simulink model "task1-1"  (R2016a)
settings: Solver=VariableStepAuto  StartTime=0.0  StopTime=10.0  RelTol=1e-3
libraries: simulink x1
settings Model: Creator=Misachu  LastModifiedBy=Misachu

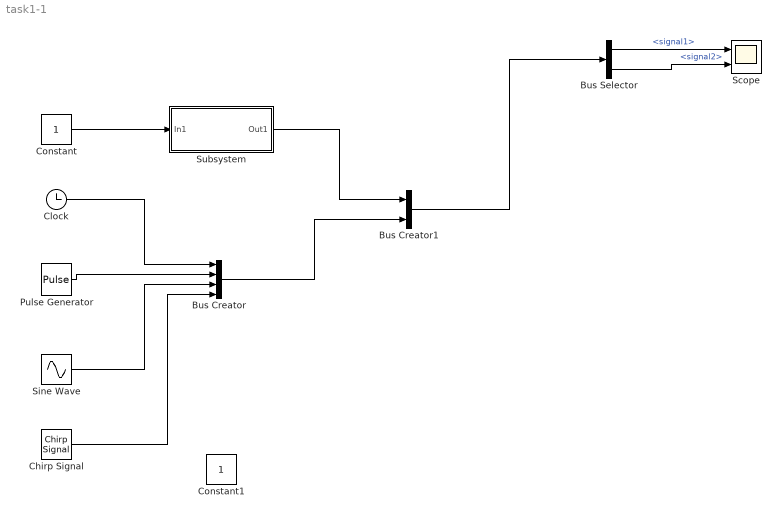
== system task1-1 ==
  Bus Creator : BusCreator  Inputs=4
  Bus Creator1 : BusCreator  Inputs=2
  Bus Selector : BusSelector  OutputSignals=signal1,signal2
  Chirp Signal : simulink/Sources/Chirp Signal  f1=0.1  T=100  f2=1
  Clock : Clock
  Constant : Constant
  Constant1 : Constant
  Pulse Generator : DiscretePulseGenerator  PulseType=Time based  Period=10  PulseWidth=5
  Scope : Scope  NumInputPorts=2
  Sine Wave : Sin  SampleTime=0
  Subsystem : Subsystem
  wires:
  Constant/1 -> Subsystem/1(In1)
  Clock/1 -> Bus Creator/1
  Pulse Generator/1 -> Bus Creator/2
  Sine Wave/1 -> Bus Creator/3
  Subsystem/1(Out1) -> Bus Creator1/1
  Bus Creator/1 -> Bus Creator1/2
  Bus Creator1/1 -> Bus Selector/1
  Bus Selector/1 -> Scope/1  "<signal1>"
  Bus Selector/2 -> Scope/2  "<signal2>"
  Chirp Signal/1 -> Bus Creator/4

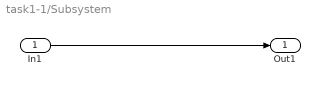
== system task1-1/Subsystem ==
  In1 : Inport
  Out1 : Outport
  wires:
  In1/1 -> Out1/1
